simulink model "Solar_PV_Module_Design"  (R2023b)
settings: Solver=VariableStepAuto  StartTime=0.0  StopTime=2.0  RelTol=1e-3
libraries: spsGroundLib x2, spsCurrentMeasurementLib x1, spsPVArrayLib x1, spsSeriesRLCBranchLib x1, spsVoltageMeasurementLib x1, spspowerguiLib x1
settings Model: Creator=HP  LastModifiedBy=HP

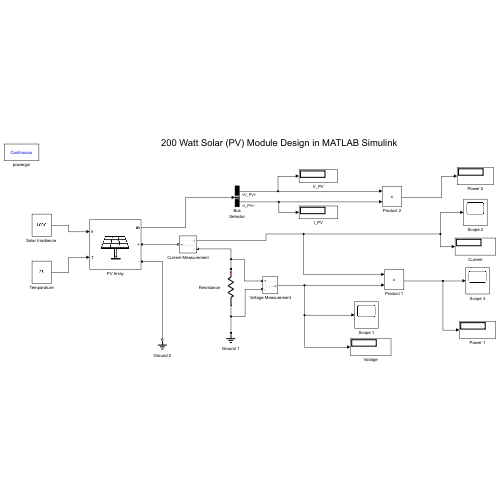
[thumbnail: Simulink's stored preview of the top-level diagram]
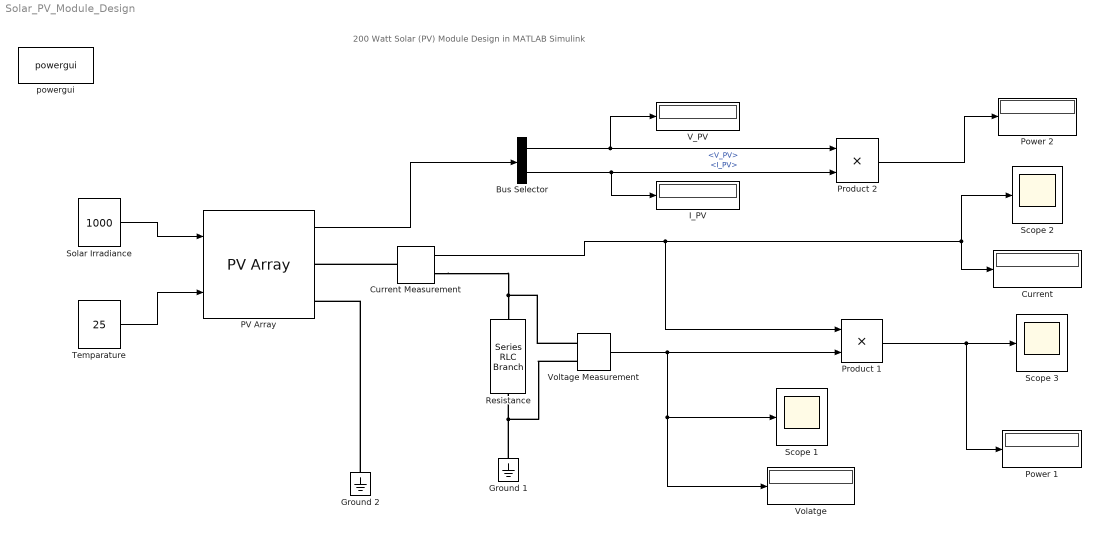
== system Solar_PV_Module_Design ==
  note: 200 Watt Solar (PV) Module Design in MATLAB Simulink
  Bus Selector : BusSelector  OutputSignals=V_PV,I_PV
  Current : Display
  Current Measurement : spsCurrentMeasurementLib/Current Measurement  PhasorSimulation=off  OutputType=Complex  PSBequivalent=0
  Ground 1 : spsGroundLib/Ground  LConnTagsString=a
  Ground 2 : spsGroundLib/Ground  LConnTagsString=a
  I_PV : Display
  PV Array : spsPVArrayLib/PV Array  Npar=1  Nser=1  PlotType=array @ 1000 W/m2 & specified temperatures  S_vec="[ 1000  500  100 ]"  Temp_C_vec="[ 45 25  ]"  ModuleName=User-defined  PlotWhenSelected=off  Pm=200.112  Ncell=60  Voc=32.9  Isc=8.21  Vm=26.4  Im=7.58  beta_Voc_pc=-0.36099  alpha_Isc_pc=0.102  beta_Voc=-0.11877  alpha_Isc=0.0083742  IL=8.2311  I0=3.0465e-10  nI=0.88972  Rsh=126.9933  Rs=0.32653  RobustModel=off  RobustCellTemperature=313.3991  BAL=on  Tc=1e-6  Tfilter=5e-5
  Power 1 : Display
  Power 2 : Display
  Product 1 : Product
  Product 2 : Product
  Resistance : spsSeriesRLCBranchLib/Series RLC Branch  LConnTagsString=__new0  RConnTagsString=__new0  BranchType=R  Resistance=3.48  Inductance=1e-3  SetiL0=off  InitialCurrent=0  Capacitance=1e-6  Setx0=off  InitialVoltage=0  Measurements=None
  Scope 1 : Scope
  Scope 2 : Scope
  Scope 3 : Scope
  "Solar Irradiance " : Constant  Value=1000
  Temparature : Constant  Value=25
  V_PV : Display
  Volatge : Display
  Voltage Measurement : spsVoltageMeasurementLib/Voltage Measurement  PhasorSimulation=off  OutputType=Complex  PSBequivalent=0
  powergui : spspowerguiLib/powergui  Priority=1  SimulationMode=Continuous  SampleTime=50e-6  frequency=60  Iterations=50  frequencyindice=0  Pbase=100e6  ErrMax=1e-4  UnitsV=kV  UnitsW=MW  buscounter=0  FunctionMessages=off  echomessages=off  EnableUseOfTLC=off  CurrentSourceSwitches=off  DisableSnubberDevices=off  DisableRonSwitches=off  DisableVfSwitches=off  DisplayEquations=off  AutomaticDiscreteSolvers=off  SolverType=Tustin/Backward Euler (TBE)  Interpol=off  ExternalGateDelay=off  methode=off  Ts=100  x0status=blocks  SPID=on  SwTol=0  HookPort=off  NonlinearTolerance=1e-4  nMaxIteration=100  ContinueOnMaxIteration=off  RestoreLinks=warning  ResistiveCurrentMeasurement=off  Frange=[0:2:500]  Ylog=off  Xlog=on  ShowGrid=off  save=off  variable=ZData  structure=0  ZoomFFT=off  StartTime=0.0  cycles=1  DisplayStyle=1  fundamental=60  FreqAxis=off  MaxFrequency=1000  frequencyindicesteady=1  RmsSteady=1  display=off
  wires:
  "Solar Irradiance "/1 -> PV Array/1
  Temparature/1 -> PV Array/2
  Voltage Measurement/1 -> Product 1/2, Scope 1/1, Volatge/1
  Current Measurement/1 -> Product 1/1, Current/1, Scope 2/1
  Product 1/1 -> Power 1/1, Scope 3/1
  PV Array/1 -> Bus Selector/1
  Bus Selector/1 -> V_PV/1, Product 2/1  "<V_PV>"
  Bus Selector/2 -> I_PV/1, Product 2/2  "<I_PV>"
  Product 2/1 -> Power 2/1
  connections:
  Ground 1/LConn1 -- Resistance/RConn1 -- Voltage Measurement/LConn2
  Current Measurement/LConn1 -- PV Array/RConn1
  Current Measurement/RConn1 -- Voltage Measurement/LConn1 -- Resistance/LConn1
  Ground 2/LConn1 -- PV Array/RConn2
